simulink model "latesttopology1"  (R2014b)
settings: Solver=ode23tb  StartTime=0.0  StopTime=1  MaxStep=0.0001  MinStep=0.00001  RelTol=1e-3
libraries: powerlib x90, simulink x33, powerlib_meascontrol x2
settings Model: Creator=SELVA  LastModifiedBy=SELVA
settings DataIOCC: SignalLoggingSaveFormat=ModelDataLogs
settings OptimizationCC: ExpressionDepthLimit=2147483647
settings DebuggingCC: UnderspecifiedInitializationDetection=Classic  MergeDetectMultiDrivingBlocksExec=none  FcnCallInpInsideContextMsg=UseLocalSettings  StateNameClashWarn=warning
settings GRTTargetCC: CombineOutputUpdateFcns=off  GRTInterface=on

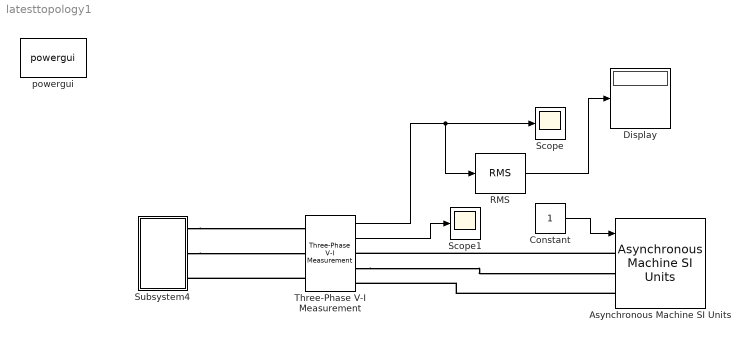
== system latesttopology1 ==
  Asynchronous Machine SI Units : powerlib/Machines/Asynchronous Machine SI Units  PresetModel="15:  5.4 HP (4KW)   400 V  50Hz 1430 RPM"  MechanicalLoad=Torque Tm  ShowDetailedParameters=on  RotorType=Squirrel-cage  ReferenceFrame=Rotor  Units=SI  MeasurementBus=off  NominalParameters=[4000 400 50]  Stator=[1.405 0.005839]  Rotor=[1.395 0.005839]  Cage1=[ 0.022 0.226/377]  Cage2=[ 0.022 0.226/377]  Lm=0.1722  Mechanical=[0.0131 0.002985 2]  PolePairs=2  InitialConditions=[1 0 0 0 0 0 0 0]  SimulateSaturation=off  Saturation=[14.03593122, 27.81365428, 53.79336849, 72.68890987, 97.98006896, 148.6815601, 215.7428561, 302.9841135, 420.4778367 ; 230, 322, 414, 460, 506, 552, 598, 644, 690]  LoadFlowParameters=1492000  TsPowergui=0  TsBlock=-1  IterativeModel=Trapezoidal non iterative  Pmec=0
  Constant : Constant
  Display : Display
  RMS : powerlib_meascontrol/Measurements/RMS  TrueRMS=on  Freq=50  RMSInit=0  Ts=0
  Scope : Scope
      settings: YMin=-800  YMax=800  SaveName=ScopeData3
  Scope1 : Scope
      settings: YMin=-800  YMax=800  SaveName=ScopeData4
  Subsystem4 : Subsystem  mask{v=66.5, fc=1000, m=1}
      mask prompts: v "DC Voltage"; fc "Switching Frequency"; m "Modulation Index"
  Three-Phase V-I Measurement : powerlib/Measurements/Three-Phase V-I Measurement  VoltageMeasurement=phase-to-ground  SetLabelV=off  LabelV=Vabc  Vpu=off  VpuLL=off  CurrentMeasurement=yes  SetLabelI=off  LabelI=Iabc  Ipu=off  Pbase=100e6  Vbase=500e3  OutputType=Complex  PhasorSimulation=off  PSBequivalent=0
  powergui : powerlib/powergui  Priority=1  SimulationMode=Discrete  SolverType=Tustin/Backward Euler (TBE)  SampleTime=50e-6  frequency=60  SPID=off  DisableSnubberDevices=off  DisableRonSwitches=off  DisableVfSwitches=off  SwTol=0  DisplayEquations=off  Interpol=off  methode=off  Ts=100  frequencyindice=0  Pbase=100e6  ErrMax=1e-4  Iterations=50  UnitsV=kV  UnitsW=MW  FunctionMessages=off  echomessages=off  HookPort=off  EnableUseOfTLC=off  x0status=blocks  RestoreLinks=warning  ResistiveCurrentMeasurement=off  Frange=[0:2:500]  Ylog=off  Xlog=on  ShowGrid=off  save=off  variable=ZData  structure=0  ZoomFFT=off  StartTime=0.0  cycles=1  DisplayStyle=1  fundamental=60  FreqAxis=off  MaxFrequency=1000  frequencyindicesteady=1  RmsSteady=1  display=off
  wires:
  Three-Phase V-I Measurement/1 -> RMS/1, Scope/1
  RMS/1 -> Display/1
  Three-Phase V-I Measurement/2 -> Scope1/1
  Constant/1 -> Asynchronous Machine SI Units/1
  connections:
  Asynchronous Machine SI Units/LConn1 -- Three-Phase V-I Measurement/RConn1
  Three-Phase V-I Measurement/RConn2 -- Asynchronous Machine SI Units/LConn2
  Asynchronous Machine SI Units/LConn3 -- Three-Phase V-I Measurement/RConn3
  Subsystem4/RConn1 -- Three-Phase V-I Measurement/LConn1
  Subsystem4/RConn2 -- Three-Phase V-I Measurement/LConn2
  Three-Phase V-I Measurement/LConn3 -- Subsystem4/RConn3

== system latesttopology1/Subsystem4 ==
  Ground : powerlib/Elements/Ground  LConnTagsString=a
  Subsystem1 : Subsystem
  Subsystem2 : Subsystem
  Subsystem3 : Subsystem
  A : PMIOPort  Port=1  Side=Right
  B : PMIOPort  Port=2  Side=Right
  C : PMIOPort  Port=3  Side=Right
  connections:
  Subsystem1/RConn2 -- Subsystem2/RConn2 -- Ground/LConn1 -- Subsystem3/RConn2
  B/RConn1 -- Subsystem2/RConn1
  A/RConn1 -- Subsystem1/RConn1
  Subsystem3/RConn1 -- C/RConn1

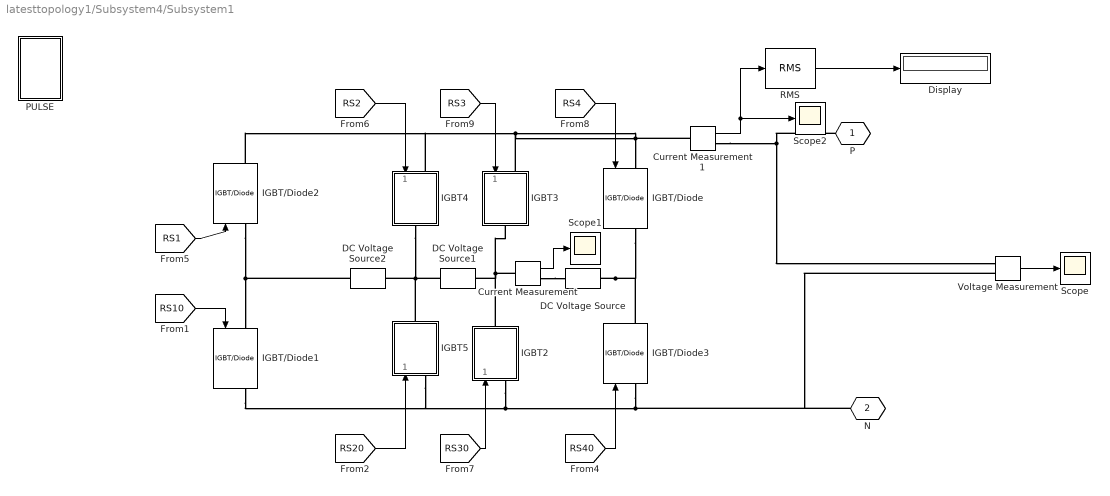
== system latesttopology1/Subsystem4/Subsystem1 ==
  Current Measurement : powerlib/Measurements/Current Measurement  PhasorSimulation=off  OutputType=Complex  PSBequivalent=0
  Current Measurement1 : powerlib/Measurements/Current Measurement  PhasorSimulation=off  OutputType=Complex  PSBequivalent=0
  DC Voltage Source : powerlib/Electrical Sources/DC Voltage Source  Amplitude=v  Measurements=None
  DC Voltage Source1 : powerlib/Electrical Sources/DC Voltage Source  Amplitude=2*v  Measurements=None
  DC Voltage Source2 : powerlib/Electrical Sources/DC Voltage Source  Amplitude=2*v  Measurements=None
  Display : Display
  IGBT/Diode{,1..3} (4 alike) : powerlib/Power Electronics/IGBT//Diode  Ron=1e-3  Rs=1e5  Cs=inf  Measurements=on
  IGBT2 : Subsystem
  IGBT3 : Subsystem
  IGBT4 : Subsystem
  IGBT5 : Subsystem
  PULSE : Subsystem
  RMS : powerlib_meascontrol/Measurements/RMS  TrueRMS=on  Freq=50  RMSInit=120  Ts=0
  Scope : Scope
      settings: YMin=-50  YMax=50  SaveName=ScopeData2
  Scope1 : Scope
      settings: YMin=-50  YMax=50  SaveName=ScopeData5
  Scope2 : Scope
      settings: YMin=-6  YMax=8  SaveName=ScopeData6
  Voltage Measurement : powerlib/Measurements/Voltage Measurement  PhasorSimulation=off  OutputType=Complex  PSBequivalent=0
  P : PMIOPort  Port=1  Side=Right
  N : PMIOPort  Port=2  Side=Right
  wires:
  Voltage Measurement/1 -> Scope/1
  [RS1] -> IGBT/Diode2/1
  [RS4] -> IGBT/Diode/1
  [RS10] -> IGBT/Diode1/1
  [RS40] -> IGBT/Diode3/1
  [RS2] -> IGBT4/1(Gate)
  [RS3] -> IGBT3/1(Gate)
  [RS20] -> IGBT5/1(Gate)
  [RS30] -> IGBT2/1(Gate)
  Current Measurement/1 -> Scope1/1
  Current Measurement1/1 -> Scope2/1, RMS/1
  RMS/1 -> Display/1
  connections:
  DC Voltage Source1/RConn1 -- IGBT4/RConn1 -- IGBT5/RConn1 -- DC Voltage Source2/LConn1
  IGBT2/RConn1 -- DC Voltage Source1/LConn1 -- Current Measurement/LConn1 -- IGBT3/RConn1
  IGBT3/LConn1 -- IGBT4/LConn1 -- IGBT/Diode2/RConn1 -- Current Measurement1/LConn1 -- IGBT/Diode/LConn1
  IGBT2/LConn1 -- IGBT5/LConn1 -- IGBT/Diode1/RConn1 -- Voltage Measurement/LConn2 -- N/RConn1 -- IGBT/Diode3/LConn1
  DC Voltage Source/LConn1 -- IGBT/Diode3/RConn1 -- IGBT/Diode/RConn1
  IGBT/Diode2/LConn1 -- DC Voltage Source2/RConn1 -- IGBT/Diode1/LConn1
  Current Measurement/RConn1 -- DC Voltage Source/RConn1
  P/RConn1 -- Current Measurement1/RConn1 -- Voltage Measurement/LConn1

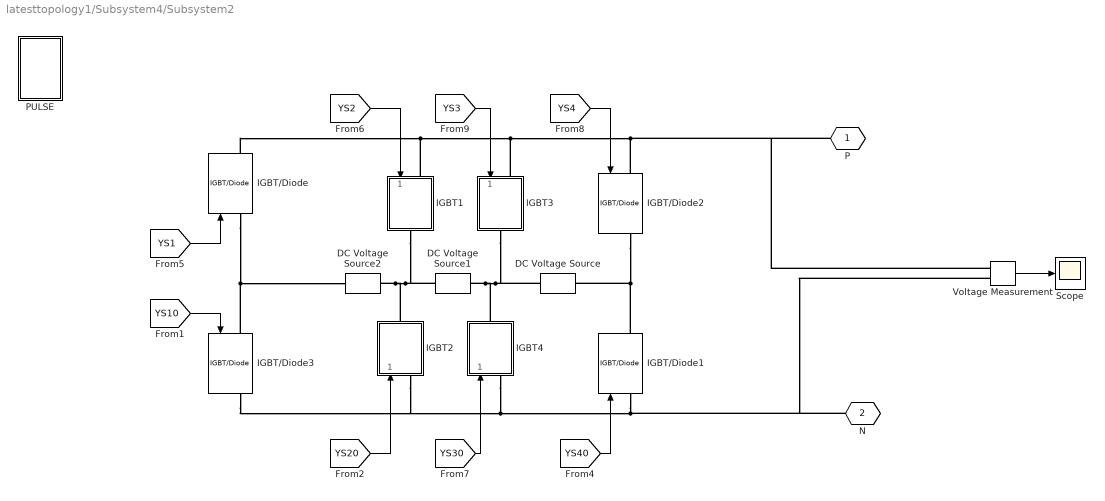
== system latesttopology1/Subsystem4/Subsystem2 ==
  DC Voltage Source : powerlib/Electrical Sources/DC Voltage Source  Amplitude=v  Measurements=None
  DC Voltage Source1 : powerlib/Electrical Sources/DC Voltage Source  Amplitude=2*v  Measurements=None
  DC Voltage Source2 : powerlib/Electrical Sources/DC Voltage Source  Amplitude=2*v  Measurements=None
  IGBT/Diode{,1..3} (4 alike) : powerlib/Power Electronics/IGBT//Diode  Ron=1e-3  Rs=1e5  Cs=inf  Measurements=on
  IGBT1 : Subsystem
  IGBT2 : Subsystem
  IGBT3 : Subsystem
  IGBT4 : Subsystem
  PULSE : Subsystem
  Scope : Scope
      settings: YMin=-50  YMax=50
  Voltage Measurement : powerlib/Measurements/Voltage Measurement  PhasorSimulation=off  OutputType=Complex  PSBequivalent=0
  P : PMIOPort  Port=1  Side=Right
  N : PMIOPort  Port=2  Side=Right
  wires:
  [YS30] -> IGBT4/1(Gate)
  [YS20] -> IGBT2/1(Gate)
  [YS3] -> IGBT3/1(Gate)
  [YS2] -> IGBT1/1(Gate)
  [YS40] -> IGBT/Diode1/1
  [YS10] -> IGBT/Diode3/1
  [YS4] -> IGBT/Diode2/1
  [YS1] -> IGBT/Diode/1
  Voltage Measurement/1 -> Scope/1
  connections:
  IGBT/Diode3/LConn1 -- IGBT/Diode/LConn1 -- DC Voltage Source2/RConn1
  IGBT/Diode2/RConn1 -- IGBT/Diode1/RConn1 -- DC Voltage Source/LConn1
  IGBT/Diode1/LConn1 -- N/RConn1 -- Voltage Measurement/LConn2 -- IGBT2/LConn1 -- IGBT/Diode3/RConn1 -- IGBT4/LConn1
  IGBT/Diode/RConn1 -- IGBT3/LConn1 -- IGBT/Diode2/LConn1 -- P/RConn1 -- Voltage Measurement/LConn1 -- IGBT1/LConn1
  DC Voltage Source1/LConn1 -- IGBT3/RConn1 -- DC Voltage Source/RConn1 -- IGBT4/RConn1
  DC Voltage Source2/LConn1 -- IGBT1/RConn1 -- DC Voltage Source1/RConn1 -- IGBT2/RConn1

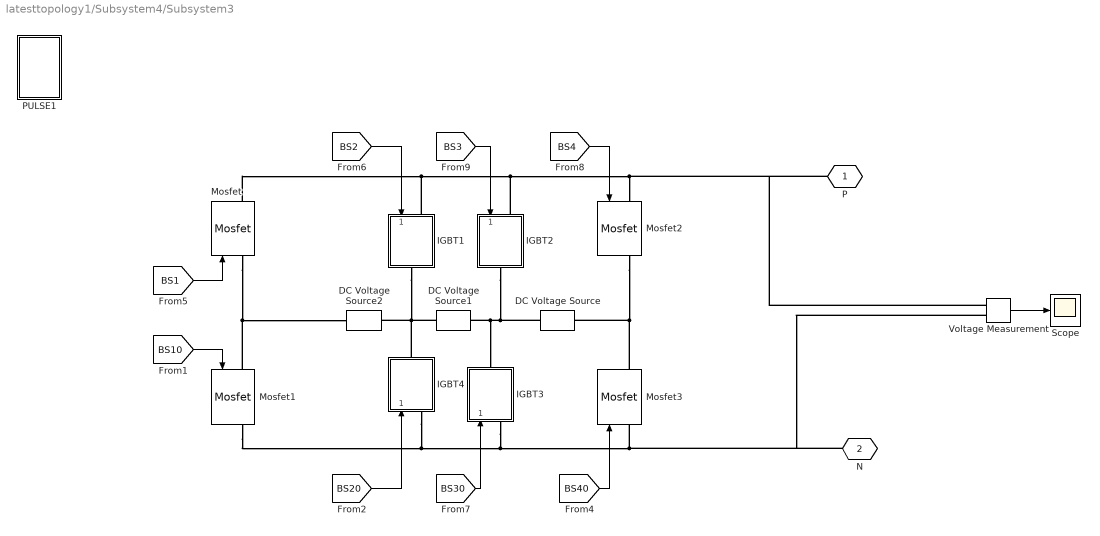
== system latesttopology1/Subsystem4/Subsystem3 ==
  DC Voltage Source : powerlib/Electrical Sources/DC Voltage Source  Amplitude=v  Measurements=None
  DC Voltage Source1 : powerlib/Electrical Sources/DC Voltage Source  Amplitude=2*v  Measurements=None
  DC Voltage Source2 : powerlib/Electrical Sources/DC Voltage Source  Amplitude=2*v  Measurements=None
  IGBT1 : Subsystem
  IGBT2 : Subsystem
  IGBT3 : Subsystem
  IGBT4 : Subsystem
  Mosfet{,1..3} (4 alike) : powerlib/Power Electronics/Mosfet  Ron=0.1  Lon=0  Rd=0.01  Vfd=0  IC=0  Rs=1e5  Cs=inf  Measurements=on
  PULSE1 : Subsystem
  Scope : Scope
      settings: YMin=-50  YMax=50
  Voltage Measurement : powerlib/Measurements/Voltage Measurement  PhasorSimulation=off  OutputType=Complex  PSBequivalent=0
  P : PMIOPort  Port=1  Side=Right
  N : PMIOPort  Port=2  Side=Right
  wires:
  Voltage Measurement/1 -> Scope/1
  [BS1] -> Mosfet/1
  [BS4] -> Mosfet2/1
  [BS10] -> Mosfet1/1
  [BS40] -> Mosfet3/1
  [BS2] -> IGBT1/1(Gate)
  [BS3] -> IGBT2/1(Gate)
  [BS20] -> IGBT4/1(Gate)
  [BS30] -> IGBT3/1(Gate)
  connections:
  IGBT4/RConn1 -- IGBT1/RConn1 -- DC Voltage Source1/RConn1 -- DC Voltage Source2/LConn1
  IGBT2/RConn1 -- DC Voltage Source/RConn1 -- IGBT3/RConn1 -- DC Voltage Source1/LConn1
  IGBT1/LConn1 -- IGBT2/LConn1 -- Voltage Measurement/LConn1 -- P/RConn1 -- Mosfet2/LConn1 -- Mosfet/RConn1
  Mosfet1/RConn1 -- IGBT4/LConn1 -- Voltage Measurement/LConn2 -- N/RConn1 -- Mosfet3/LConn1 -- IGBT3/LConn1
  Mosfet2/RConn1 -- DC Voltage Source/LConn1 -- Mosfet3/RConn1
  Mosfet/LConn1 -- Mosfet1/LConn1 -- DC Voltage Source2/RConn1

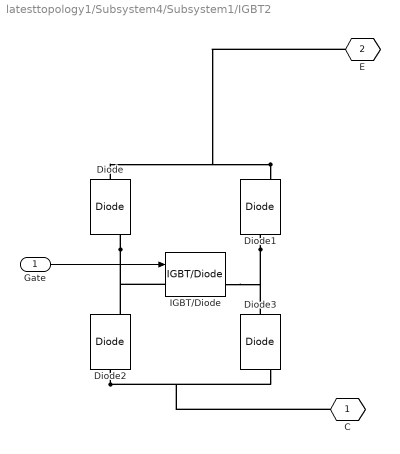
== system latesttopology1/Subsystem4/Subsystem1/IGBT2 ==
  Gate : Inport
  Diode{,1..3} (4 alike) : powerlib/Power Electronics/Diode  Ron=0.001  Lon=0  Vf=0.8  IC=0  UseSnubber=off  Rs=500  Cs=250e-9  Measurements=on
  IGBT/Diode : powerlib/Power Electronics/IGBT//Diode  Ron=1e-3  Rs=1e5  Cs=inf  Measurements=on
  C : PMIOPort  Port=1  Side=Left
  E : PMIOPort  Port=2  Side=Right
  wires:
  Gate/1 -> IGBT/Diode/1
  connections:
  Diode/RConn1 -- Diode2/RConn1 -- IGBT/Diode/LConn1
  Diode1/LConn1 -- Diode3/LConn1 -- IGBT/Diode/RConn1
  Diode2/LConn1 -- Diode3/RConn1 -- C/RConn1
  Diode1/RConn1 -- Diode/LConn1 -- E/RConn1

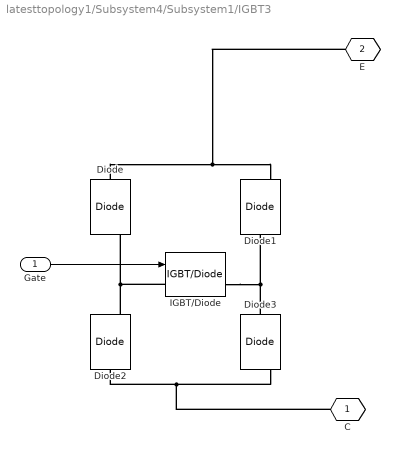
== system latesttopology1/Subsystem4/Subsystem1/IGBT3 ==
  Gate : Inport
  Diode{,1..3} (4 alike) : powerlib/Power Electronics/Diode  Ron=0.001  Lon=0  Vf=0.8  IC=0  UseSnubber=off  Rs=500  Cs=250e-9  Measurements=on
  IGBT/Diode : powerlib/Power Electronics/IGBT//Diode  Ron=1e-3  Rs=1e5  Cs=inf  Measurements=on
  C : PMIOPort  Port=1  Side=Left
  E : PMIOPort  Port=2  Side=Right
  wires:
  Gate/1 -> IGBT/Diode/1
  connections:
  E/RConn1 -- Diode/LConn1 -- Diode1/RConn1
  C/RConn1 -- Diode3/RConn1 -- Diode2/LConn1
  IGBT/Diode/RConn1 -- Diode3/LConn1 -- Diode1/LConn1
  IGBT/Diode/LConn1 -- Diode2/RConn1 -- Diode/RConn1

== system latesttopology1/Subsystem4/Subsystem1/IGBT4 ==
  Gate : Inport
  Diode{,1..3} (4 alike) : powerlib/Power Electronics/Diode  Ron=0.001  Lon=0  Vf=0.8  IC=0  UseSnubber=off  Rs=500  Cs=250e-9  Measurements=on
  IGBT/Diode : powerlib/Power Electronics/IGBT//Diode  Ron=1e-3  Rs=1e5  Cs=inf  Measurements=on
  C : PMIOPort  Port=1  Side=Left
  E : PMIOPort  Port=2  Side=Right
  wires:
  Gate/1 -> IGBT/Diode/1
  connections:
  Diode/RConn1 -- Diode2/RConn1 -- IGBT/Diode/LConn1
  Diode1/LConn1 -- Diode3/LConn1 -- IGBT/Diode/RConn1
  Diode2/LConn1 -- Diode3/RConn1 -- C/RConn1
  Diode1/RConn1 -- Diode/LConn1 -- E/RConn1

== system latesttopology1/Subsystem4/Subsystem1/IGBT5 ==
  Gate : Inport
  Diode{,1..3} (4 alike) : powerlib/Power Electronics/Diode  Ron=0.001  Lon=0  Vf=0.8  IC=0  UseSnubber=off  Rs=500  Cs=250e-9  Measurements=on
  IGBT/Diode : powerlib/Power Electronics/IGBT//Diode  Ron=1e-3  Rs=1e5  Cs=inf  Measurements=on
  C : PMIOPort  Port=1  Side=Left
  E : PMIOPort  Port=2  Side=Right
  wires:
  Gate/1 -> IGBT/Diode/1
  connections:
  E/RConn1 -- Diode/LConn1 -- Diode1/RConn1
  C/RConn1 -- Diode3/RConn1 -- Diode2/LConn1
  IGBT/Diode/RConn1 -- Diode3/LConn1 -- Diode1/LConn1
  IGBT/Diode/LConn1 -- Diode2/RConn1 -- Diode/RConn1

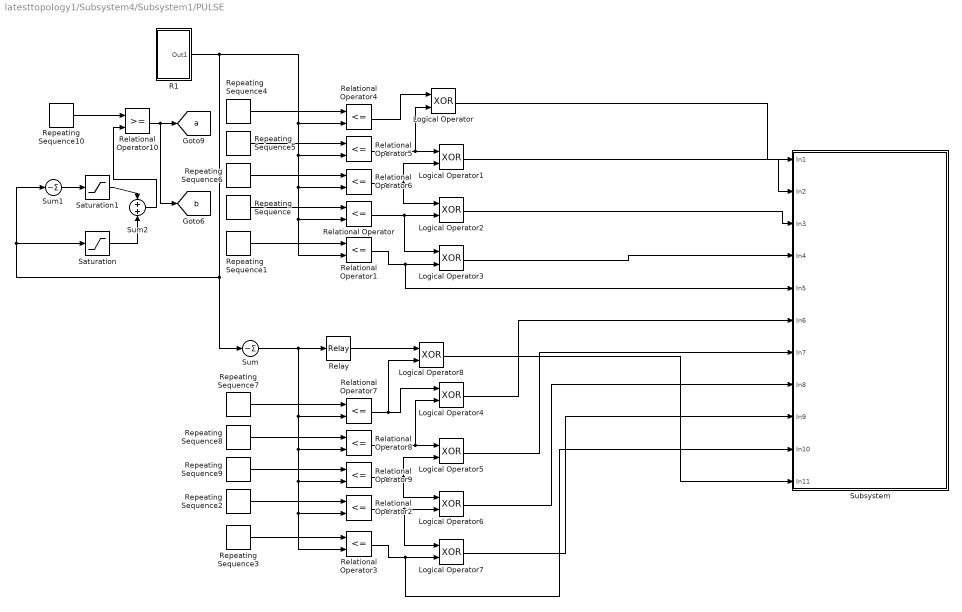
== system latesttopology1/Subsystem4/Subsystem1/PULSE ==
  Logical Operator{,1..8} (9 alike) : Logic  Operator=XOR  AllPortsSameDT=off  OutDataTypeStr=boolean
  R1 : Subsystem
  Relational Operator{,1..9} (10 alike) : RelationalOperator  Operator=<=  OutDataTypeStr=boolean
  Relational Operator10 : RelationalOperator  OutDataTypeStr=boolean
  Relay : Relay  OnOutputValue=0  OffOutputValue=1
  Repeating Sequence : simulink/Sources/Repeating Sequence  rep_seq_t="[0 (1/fc)/2  (1/fc)]"  rep_seq_y=[3/5 4/5 3/5]
  Repeating Sequence1 : simulink/Sources/Repeating Sequence  rep_seq_t="[0 (1/fc)/2  (1/fc)]"  rep_seq_y=[4/5 1 4/5]
  Repeating Sequence10 : simulink/Sources/Repeating Sequence  rep_seq_t="[0 (1/fc)/2  (1/fc)]"  rep_seq_y=[0 1/5 0]
  Repeating Sequence2 : simulink/Sources/Repeating Sequence  rep_seq_t="[0 (1/fc)/2  (1/fc)]"  rep_seq_y=[3/5 4/5 3/5]
  Repeating Sequence3 : simulink/Sources/Repeating Sequence  rep_seq_t="[0 (1/fc)/2  (1/fc)]"  rep_seq_y=[4/5 1 4/5]
  Repeating Sequence4 : simulink/Sources/Repeating Sequence  rep_seq_t="[0 (1/fc)/2  (1/fc)]"  rep_seq_y=[0 1/5 0]
  Repeating Sequence5 : simulink/Sources/Repeating Sequence  rep_seq_t="[0 (1/fc)/2  (1/fc)]"  rep_seq_y=[1/5 2/5 1/5]
  Repeating Sequence6 : simulink/Sources/Repeating Sequence  rep_seq_t="[0 (1/fc)/2  (1/fc)]"  rep_seq_y=[2/5 3/5 2/5]
  Repeating Sequence7 : simulink/Sources/Repeating Sequence  rep_seq_t="[0 (1/fc)/2  (1/fc)]"  rep_seq_y=[0 1/5 0]
  Repeating Sequence8 : simulink/Sources/Repeating Sequence  rep_seq_t="[0 (1/fc)/2  (1/fc)]"  rep_seq_y=[1/5 2/5 1/5]
  Repeating Sequence9 : simulink/Sources/Repeating Sequence  rep_seq_t="[0 (1/fc)/2  (1/fc)]"  rep_seq_y=[2/5 3/5 2/5]
  Saturation : Saturate  UpperLimit=1  LowerLimit=0
  Saturation1 : Saturate  UpperLimit=1  LowerLimit=0
  Subsystem : Subsystem
  Sum : Sum  Inputs=-
  Sum1 : Sum  Inputs=-
  Sum2 : Sum
  tag scope: a=global, b=global
  wires:
  Repeating Sequence1/1 -> Relational Operator1/1
  Repeating Sequence/1 -> Relational Operator/1
  Repeating Sequence6/1 -> Relational Operator6/1
  Repeating Sequence5/1 -> Relational Operator5/1
  Repeating Sequence4/1 -> Relational Operator4/1
  R1/1(Out1) -> Sum1/1, Saturation/1, Sum/1, Relational Operator4/2, Relational Operator5/2, Relational Operator6/2, Relational Operator1/2, Relational Operator/2
  Relational Operator4/1 -> Logical Operator/1
  Relational Operator5/1 -> Logical Operator1/1, Logical Operator/2
  Relational Operator6/1 -> Logical Operator2/1, Logical Operator1/2
  Relational Operator/1 -> Logical Operator3/1, Logical Operator2/2
  Relational Operator1/1 -> Subsystem/5(In5), Logical Operator3/2
  Repeating Sequence3/1 -> Relational Operator3/1
  Repeating Sequence2/1 -> Relational Operator2/1
  Repeating Sequence9/1 -> Relational Operator9/1
  Repeating Sequence8/1 -> Relational Operator8/1
  Repeating Sequence7/1 -> Relational Operator7/1
  Sum/1 -> Relay/1, Relational Operator7/2, Relational Operator8/2, Relational Operator9/2, Relational Operator3/2, Relational Operator2/2
  Relational Operator7/1 -> Logical Operator8/2, Logical Operator4/1
  Relational Operator8/1 -> Logical Operator5/1, Logical Operator4/2
  Relational Operator9/1 -> Logical Operator6/1, Logical Operator5/2
  Relational Operator2/1 -> Logical Operator7/1, Logical Operator6/2
  Relational Operator3/1 -> Subsystem/10(In10), Logical Operator7/2
  Logical Operator4/1 -> Subsystem/6(In6)
  Logical Operator6/1 -> Subsystem/8(In8)
  Logical Operator7/1 -> Subsystem/9(In9)
  Logical Operator/1 -> Subsystem/1(In1)
  Logical Operator1/1 -> Subsystem/2(In2)
  Logical Operator2/1 -> Subsystem/3(In3)
  Logical Operator3/1 -> Subsystem/4(In4)
  Logical Operator5/1 -> Subsystem/7(In7)
  Relay/1 -> Logical Operator8/1
  Logical Operator8/1 -> Subsystem/11(In11)
  Sum1/1 -> Saturation1/1
  Saturation1/1 -> Sum2/1
  Saturation/1 -> Sum2/2
  Repeating Sequence10/1 -> Relational Operator10/1
  Sum2/1 -> Relational Operator10/2
  Relational Operator10/1 -> [b], [a]

== system latesttopology1/Subsystem4/Subsystem2/IGBT1 ==
  Gate : Inport
  Diode{,1..3} (4 alike) : powerlib/Power Electronics/Diode  Ron=0.001  Lon=0  Vf=0.8  IC=0  UseSnubber=off  Rs=500  Cs=250e-9  Measurements=on
  IGBT/Diode : powerlib/Power Electronics/IGBT//Diode  Ron=1e-3  Rs=1e5  Cs=inf  Measurements=on
  C : PMIOPort  Port=1  Side=Left
  E : PMIOPort  Port=2  Side=Right
  wires:
  Gate/1 -> IGBT/Diode/1
  connections:
  Diode/RConn1 -- Diode2/RConn1 -- IGBT/Diode/LConn1
  Diode1/LConn1 -- Diode3/LConn1 -- IGBT/Diode/RConn1
  Diode2/LConn1 -- Diode3/RConn1 -- C/RConn1
  Diode1/RConn1 -- Diode/LConn1 -- E/RConn1

== system latesttopology1/Subsystem4/Subsystem2/IGBT2 ==
  Gate : Inport
  Diode{,1..3} (4 alike) : powerlib/Power Electronics/Diode  Ron=0.001  Lon=0  Vf=0.8  IC=0  UseSnubber=off  Rs=500  Cs=250e-9  Measurements=on
  IGBT/Diode : powerlib/Power Electronics/IGBT//Diode  Ron=1e-3  Rs=1e5  Cs=inf  Measurements=on
  C : PMIOPort  Port=1  Side=Left
  E : PMIOPort  Port=2  Side=Right
  wires:
  Gate/1 -> IGBT/Diode/1
  connections:
  E/RConn1 -- Diode/LConn1 -- Diode1/RConn1
  C/RConn1 -- Diode3/RConn1 -- Diode2/LConn1
  IGBT/Diode/RConn1 -- Diode3/LConn1 -- Diode1/LConn1
  IGBT/Diode/LConn1 -- Diode2/RConn1 -- Diode/RConn1

== system latesttopology1/Subsystem4/Subsystem2/IGBT3 ==
  Gate : Inport
  Diode{,1..3} (4 alike) : powerlib/Power Electronics/Diode  Ron=0.001  Lon=0  Vf=0.8  IC=0  UseSnubber=off  Rs=500  Cs=250e-9  Measurements=on
  IGBT/Diode : powerlib/Power Electronics/IGBT//Diode  Ron=1e-3  Rs=1e5  Cs=inf  Measurements=on
  C : PMIOPort  Port=1  Side=Left
  E : PMIOPort  Port=2  Side=Right
  wires:
  Gate/1 -> IGBT/Diode/1
  connections:
  E/RConn1 -- Diode/LConn1 -- Diode1/RConn1
  C/RConn1 -- Diode3/RConn1 -- Diode2/LConn1
  IGBT/Diode/RConn1 -- Diode3/LConn1 -- Diode1/LConn1
  IGBT/Diode/LConn1 -- Diode2/RConn1 -- Diode/RConn1

== system latesttopology1/Subsystem4/Subsystem2/IGBT4 ==
  Gate : Inport
  Diode{,1..3} (4 alike) : powerlib/Power Electronics/Diode  Ron=0.001  Lon=0  Vf=0.8  IC=0  UseSnubber=off  Rs=500  Cs=250e-9  Measurements=on
  IGBT/Diode : powerlib/Power Electronics/IGBT//Diode  Ron=1e-3  Rs=1e5  Cs=inf  Measurements=on
  C : PMIOPort  Port=1  Side=Left
  E : PMIOPort  Port=2  Side=Right
  wires:
  Gate/1 -> IGBT/Diode/1
  connections:
  Diode/RConn1 -- Diode2/RConn1 -- IGBT/Diode/LConn1
  Diode1/LConn1 -- Diode3/LConn1 -- IGBT/Diode/RConn1
  Diode2/LConn1 -- Diode3/RConn1 -- C/RConn1
  Diode1/RConn1 -- Diode/LConn1 -- E/RConn1

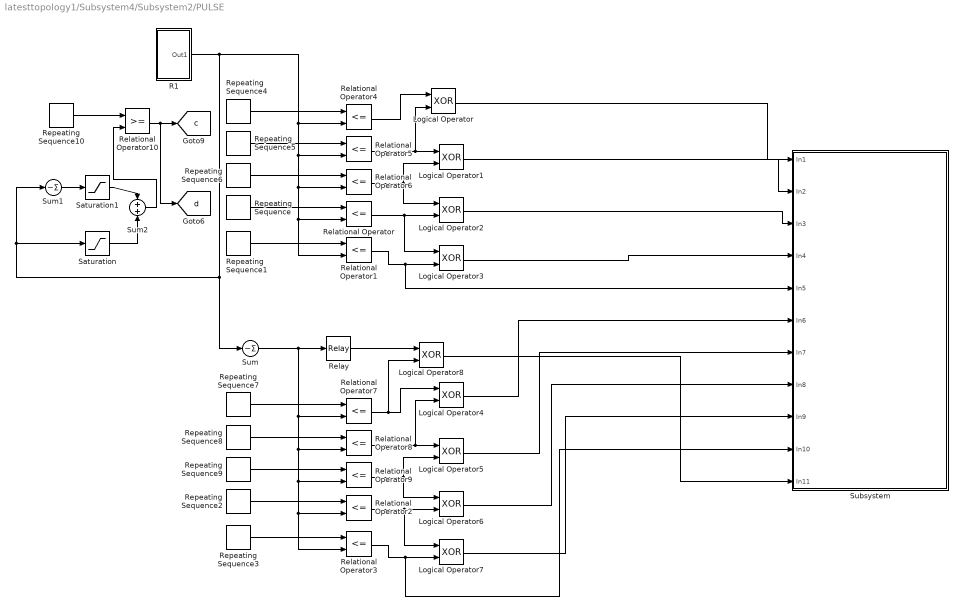
== system latesttopology1/Subsystem4/Subsystem2/PULSE ==
  Logical Operator{,1..8} (9 alike) : Logic  Operator=XOR  AllPortsSameDT=off  OutDataTypeStr=boolean
  R1 : Subsystem
  Relational Operator{,1..9} (10 alike) : RelationalOperator  Operator=<=  OutDataTypeStr=boolean
  Relational Operator10 : RelationalOperator  OutDataTypeStr=boolean
  Relay : Relay  OnOutputValue=0  OffOutputValue=1
  Repeating Sequence : simulink/Sources/Repeating Sequence  rep_seq_t="[0 (1/fc)/2  (1/fc)]"  rep_seq_y=[3/5 4/5 3/5]
  Repeating Sequence1 : simulink/Sources/Repeating Sequence  rep_seq_t="[0 (1/fc)/2  (1/fc)]"  rep_seq_y=[4/5 1 4/5]
  Repeating Sequence10 : simulink/Sources/Repeating Sequence  rep_seq_t="[0 (1/fc)/2  (1/fc)]"  rep_seq_y=[0 1/5 0]
  Repeating Sequence2 : simulink/Sources/Repeating Sequence  rep_seq_t="[0 (1/fc)/2  (1/fc)]"  rep_seq_y=[3/5 4/5 3/5]
  Repeating Sequence3 : simulink/Sources/Repeating Sequence  rep_seq_t="[0 (1/fc)/2  (1/fc)]"  rep_seq_y=[4/5 1 4/5]
  Repeating Sequence4 : simulink/Sources/Repeating Sequence  rep_seq_t="[0 (1/fc)/2  (1/fc)]"  rep_seq_y=[0 1/5 0]
  Repeating Sequence5 : simulink/Sources/Repeating Sequence  rep_seq_t="[0 (1/fc)/2  (1/fc)]"  rep_seq_y=[1/5 2/5 1/5]
  Repeating Sequence6 : simulink/Sources/Repeating Sequence  rep_seq_t="[0 (1/fc)/2  (1/fc)]"  rep_seq_y=[2/5 3/5 2/5]
  Repeating Sequence7 : simulink/Sources/Repeating Sequence  rep_seq_t="[0 (1/fc)/2  (1/fc)]"  rep_seq_y=[0 1/5 0]
  Repeating Sequence8 : simulink/Sources/Repeating Sequence  rep_seq_t="[0 (1/fc)/2  (1/fc)]"  rep_seq_y=[1/5 2/5 1/5]
  Repeating Sequence9 : simulink/Sources/Repeating Sequence  rep_seq_t="[0 (1/fc)/2  (1/fc)]"  rep_seq_y=[2/5 3/5 2/5]
  Saturation : Saturate  UpperLimit=1  LowerLimit=0
  Saturation1 : Saturate  UpperLimit=1  LowerLimit=0
  Subsystem : Subsystem
  Sum : Sum  Inputs=-
  Sum1 : Sum  Inputs=-
  Sum2 : Sum
  tag scope: c=global, d=global
  wires:
  Relational Operator10/1 -> [c], [d]
  Sum2/1 -> Relational Operator10/2
  Repeating Sequence10/1 -> Relational Operator10/1
  Saturation/1 -> Sum2/2
  Saturation1/1 -> Sum2/1
  Sum1/1 -> Saturation1/1
  Logical Operator8/1 -> Subsystem/11(In11)
  Relay/1 -> Logical Operator8/1
  Logical Operator5/1 -> Subsystem/7(In7)
  Logical Operator3/1 -> Subsystem/4(In4)
  Logical Operator2/1 -> Subsystem/3(In3)
  Logical Operator1/1 -> Subsystem/2(In2)
  Logical Operator/1 -> Subsystem/1(In1)
  Logical Operator7/1 -> Subsystem/9(In9)
  Logical Operator6/1 -> Subsystem/8(In8)
  Logical Operator4/1 -> Subsystem/6(In6)
  Relational Operator3/1 -> Logical Operator7/2, Subsystem/10(In10)
  Relational Operator2/1 -> Logical Operator6/2, Logical Operator7/1
  Relational Operator9/1 -> Logical Operator5/2, Logical Operator6/1
  Relational Operator8/1 -> Logical Operator4/2, Logical Operator5/1
  Relational Operator7/1 -> Logical Operator4/1, Logical Operator8/2
  Sum/1 -> Relational Operator2/2, Relational Operator3/2, Relational Operator9/2, Relational Operator8/2, Relational Operator7/2, Relay/1
  Repeating Sequence7/1 -> Relational Operator7/1
  Repeating Sequence8/1 -> Relational Operator8/1
  Repeating Sequence9/1 -> Relational Operator9/1
  Repeating Sequence2/1 -> Relational Operator2/1
  Repeating Sequence3/1 -> Relational Operator3/1
  Relational Operator1/1 -> Logical Operator3/2, Subsystem/5(In5)
  Relational Operator/1 -> Logical Operator2/2, Logical Operator3/1
  Relational Operator6/1 -> Logical Operator1/2, Logical Operator2/1
  Relational Operator5/1 -> Logical Operator/2, Logical Operator1/1
  Relational Operator4/1 -> Logical Operator/1
  R1/1(Out1) -> Relational Operator/2, Relational Operator1/2, Relational Operator6/2, Relational Operator5/2, Relational Operator4/2, Sum/1, Saturation/1, Sum1/1
  Repeating Sequence4/1 -> Relational Operator4/1
  Repeating Sequence5/1 -> Relational Operator5/1
  Repeating Sequence6/1 -> Relational Operator6/1
  Repeating Sequence/1 -> Relational Operator/1
  Repeating Sequence1/1 -> Relational Operator1/1

== system latesttopology1/Subsystem4/Subsystem3/IGBT1 ==
  Gate : Inport
  Diode{,1..3} (4 alike) : powerlib/Power Electronics/Diode  Ron=0.001  Lon=0  Vf=0.8  IC=0  UseSnubber=off  Rs=500  Cs=250e-9  Measurements=on
  IGBT/Diode : powerlib/Power Electronics/IGBT//Diode  Ron=1e-3  Rs=1e5  Cs=inf  Measurements=on
  C : PMIOPort  Port=1  Side=Left
  E : PMIOPort  Port=2  Side=Right
  wires:
  Gate/1 -> IGBT/Diode/1
  connections:
  E/RConn1 -- Diode/LConn1 -- Diode1/RConn1
  C/RConn1 -- Diode3/RConn1 -- Diode2/LConn1
  IGBT/Diode/RConn1 -- Diode3/LConn1 -- Diode1/LConn1
  IGBT/Diode/LConn1 -- Diode2/RConn1 -- Diode/RConn1

== system latesttopology1/Subsystem4/Subsystem3/IGBT2 ==
  Gate : Inport
  Diode{,1..3} (4 alike) : powerlib/Power Electronics/Diode  Ron=0.001  Lon=0  Vf=0.8  IC=0  UseSnubber=off  Rs=500  Cs=250e-9  Measurements=on
  IGBT/Diode : powerlib/Power Electronics/IGBT//Diode  Ron=1e-3  Rs=1e5  Cs=inf  Measurements=on
  C : PMIOPort  Port=1  Side=Left
  E : PMIOPort  Port=2  Side=Right
  wires:
  Gate/1 -> IGBT/Diode/1
  connections:
  Diode/RConn1 -- Diode2/RConn1 -- IGBT/Diode/LConn1
  Diode1/LConn1 -- Diode3/LConn1 -- IGBT/Diode/RConn1
  Diode2/LConn1 -- Diode3/RConn1 -- C/RConn1
  Diode1/RConn1 -- Diode/LConn1 -- E/RConn1

== system latesttopology1/Subsystem4/Subsystem3/IGBT3 ==
  Gate : Inport
  Diode{,1..3} (4 alike) : powerlib/Power Electronics/Diode  Ron=0.001  Lon=0  Vf=0.8  IC=0  UseSnubber=off  Rs=500  Cs=250e-9  Measurements=on
  IGBT/Diode : powerlib/Power Electronics/IGBT//Diode  Ron=1e-3  Rs=1e5  Cs=inf  Measurements=on
  C : PMIOPort  Port=1  Side=Left
  E : PMIOPort  Port=2  Side=Right
  wires:
  Gate/1 -> IGBT/Diode/1
  connections:
  E/RConn1 -- Diode/LConn1 -- Diode1/RConn1
  C/RConn1 -- Diode3/RConn1 -- Diode2/LConn1
  IGBT/Diode/RConn1 -- Diode3/LConn1 -- Diode1/LConn1
  IGBT/Diode/LConn1 -- Diode2/RConn1 -- Diode/RConn1

== system latesttopology1/Subsystem4/Subsystem3/IGBT4 ==
  Gate : Inport
  Diode{,1..3} (4 alike) : powerlib/Power Electronics/Diode  Ron=0.001  Lon=0  Vf=0.8  IC=0  UseSnubber=off  Rs=500  Cs=250e-9  Measurements=on
  IGBT/Diode : powerlib/Power Electronics/IGBT//Diode  Ron=1e-3  Rs=1e5  Cs=inf  Measurements=on
  C : PMIOPort  Port=1  Side=Left
  E : PMIOPort  Port=2  Side=Right
  wires:
  Gate/1 -> IGBT/Diode/1
  connections:
  Diode/RConn1 -- Diode2/RConn1 -- IGBT/Diode/LConn1
  Diode1/LConn1 -- Diode3/LConn1 -- IGBT/Diode/RConn1
  Diode2/LConn1 -- Diode3/RConn1 -- C/RConn1
  Diode1/RConn1 -- Diode/LConn1 -- E/RConn1

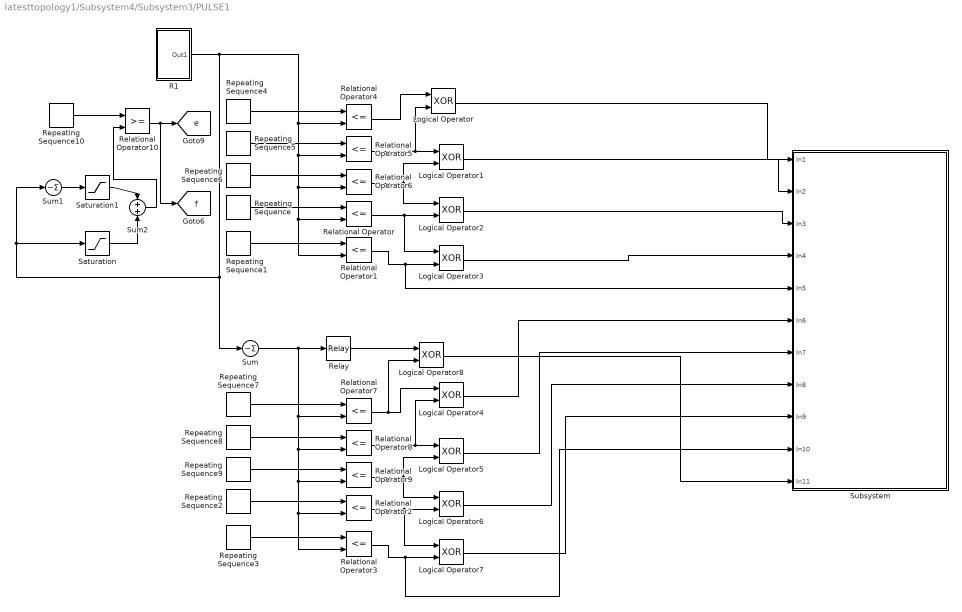
== system latesttopology1/Subsystem4/Subsystem3/PULSE1 ==
  Logical Operator{,1..8} (9 alike) : Logic  Operator=XOR  AllPortsSameDT=off  OutDataTypeStr=boolean
  R1 : Subsystem
  Relational Operator{,1..9} (10 alike) : RelationalOperator  Operator=<=  OutDataTypeStr=boolean
  Relational Operator10 : RelationalOperator  OutDataTypeStr=boolean
  Relay : Relay  OnOutputValue=0  OffOutputValue=1
  Repeating Sequence : simulink/Sources/Repeating Sequence  rep_seq_t="[0 (1/fc)/2  (1/fc)]"  rep_seq_y=[3/5 4/5 3/5]
  Repeating Sequence1 : simulink/Sources/Repeating Sequence  rep_seq_t="[0 (1/fc)/2  (1/fc)]"  rep_seq_y=[4/5 1 4/5]
  Repeating Sequence10 : simulink/Sources/Repeating Sequence  rep_seq_t="[0 (1/fc)/2  (1/fc)]"  rep_seq_y=[0 1/5 0]
  Repeating Sequence2 : simulink/Sources/Repeating Sequence  rep_seq_t="[0 (1/fc)/2  (1/fc)]"  rep_seq_y=[3/5 4/5 3/5]
  Repeating Sequence3 : simulink/Sources/Repeating Sequence  rep_seq_t="[0 (1/fc)/2  (1/fc)]"  rep_seq_y=[4/5 1 4/5]
  Repeating Sequence4 : simulink/Sources/Repeating Sequence  rep_seq_t="[0 (1/fc)/2  (1/fc)]"  rep_seq_y=[0 1/5 0]
  Repeating Sequence5 : simulink/Sources/Repeating Sequence  rep_seq_t="[0 (1/fc)/2  (1/fc)]"  rep_seq_y=[1/5 2/5 1/5]
  Repeating Sequence6 : simulink/Sources/Repeating Sequence  rep_seq_t="[0 (1/fc)/2  (1/fc)]"  rep_seq_y=[2/5 3/5 2/5]
  Repeating Sequence7 : simulink/Sources/Repeating Sequence  rep_seq_t="[0 (1/fc)/2  (1/fc)]"  rep_seq_y=[0 1/5 0]
  Repeating Sequence8 : simulink/Sources/Repeating Sequence  rep_seq_t="[0 (1/fc)/2  (1/fc)]"  rep_seq_y=[1/5 2/5 1/5]
  Repeating Sequence9 : simulink/Sources/Repeating Sequence  rep_seq_t="[0 (1/fc)/2  (1/fc)]"  rep_seq_y=[2/5 3/5 2/5]
  Saturation : Saturate  UpperLimit=1  LowerLimit=0
  Saturation1 : Saturate  UpperLimit=1  LowerLimit=0
  Subsystem : Subsystem
  Sum : Sum  Inputs=-
  Sum1 : Sum  Inputs=-
  Sum2 : Sum
  tag scope: e=global, f=global
  wires:
  Relational Operator10/1 -> [e], [f]
  Sum2/1 -> Relational Operator10/2
  Repeating Sequence10/1 -> Relational Operator10/1
  Saturation/1 -> Sum2/2
  Saturation1/1 -> Sum2/1
  Sum1/1 -> Saturation1/1
  Logical Operator8/1 -> Subsystem/11(In11)
  Relay/1 -> Logical Operator8/1
  Logical Operator5/1 -> Subsystem/7(In7)
  Logical Operator3/1 -> Subsystem/4(In4)
  Logical Operator2/1 -> Subsystem/3(In3)
  Logical Operator1/1 -> Subsystem/2(In2)
  Logical Operator/1 -> Subsystem/1(In1)
  Logical Operator7/1 -> Subsystem/9(In9)
  Logical Operator6/1 -> Subsystem/8(In8)
  Logical Operator4/1 -> Subsystem/6(In6)
  Relational Operator3/1 -> Logical Operator7/2, Subsystem/10(In10)
  Relational Operator2/1 -> Logical Operator6/2, Logical Operator7/1
  Relational Operator9/1 -> Logical Operator5/2, Logical Operator6/1
  Relational Operator8/1 -> Logical Operator4/2, Logical Operator5/1
  Relational Operator7/1 -> Logical Operator4/1, Logical Operator8/2
  Sum/1 -> Relational Operator2/2, Relational Operator3/2, Relational Operator9/2, Relational Operator8/2, Relational Operator7/2, Relay/1
  Repeating Sequence7/1 -> Relational Operator7/1
  Repeating Sequence8/1 -> Relational Operator8/1
  Repeating Sequence9/1 -> Relational Operator9/1
  Repeating Sequence2/1 -> Relational Operator2/1
  Repeating Sequence3/1 -> Relational Operator3/1
  Relational Operator1/1 -> Logical Operator3/2, Subsystem/5(In5)
  Relational Operator/1 -> Logical Operator2/2, Logical Operator3/1
  Relational Operator6/1 -> Logical Operator1/2, Logical Operator2/1
  Relational Operator5/1 -> Logical Operator/2, Logical Operator1/1
  Relational Operator4/1 -> Logical Operator/1
  R1/1(Out1) -> Relational Operator/2, Relational Operator1/2, Relational Operator6/2, Relational Operator5/2, Relational Operator4/2, Sum/1, Saturation/1, Sum1/1
  Repeating Sequence4/1 -> Relational Operator4/1
  Repeating Sequence5/1 -> Relational Operator5/1
  Repeating Sequence6/1 -> Relational Operator6/1
  Repeating Sequence/1 -> Relational Operator/1
  Repeating Sequence1/1 -> Relational Operator1/1

== system latesttopology1/Subsystem4/Subsystem1/PULSE/R1 ==
  Sine Wave : Sin  Amplitude=m  Frequency=2*pi*50  SampleTime=0
  Out1 : Outport
  wires:
  Sine Wave/1 -> Out1/1

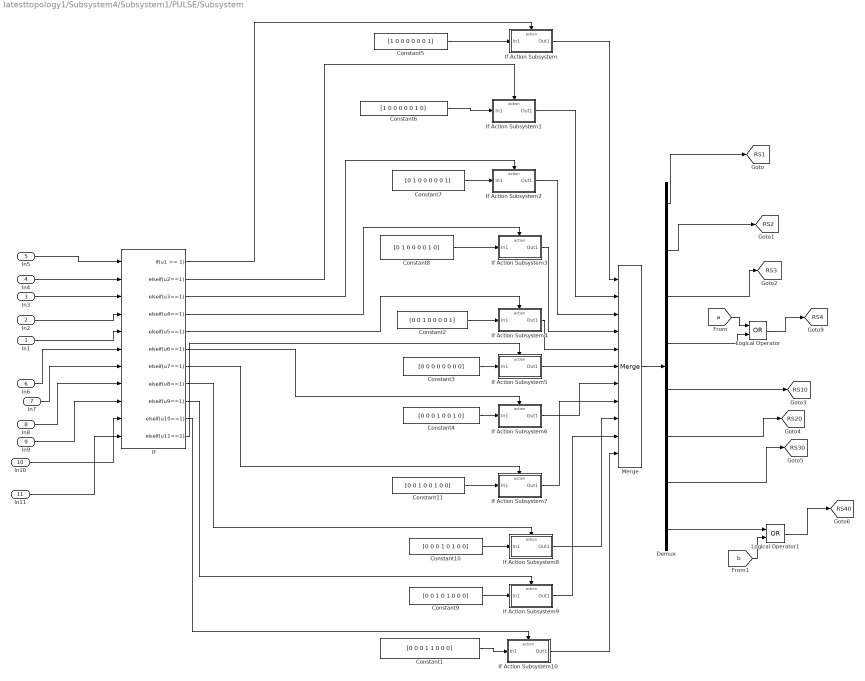
== system latesttopology1/Subsystem4/Subsystem1/PULSE/Subsystem ==
  In1 : Inport
  In2 : Inport  Port=2
  In3 : Inport  Port=3
  In4 : Inport  Port=4
  In5 : Inport  Port=5
  In6 : Inport  Port=6
  In7 : Inport  Port=7
  In8 : Inport  Port=8
  In9 : Inport  Port=9
  In10 : Inport  Port=10
  In11 : Inport  Port=11
  Constant1 : Constant  Value=[0 0 0 1 1 0 0 0]
  Constant10 : Constant  Value=[0 0 0 1 0 1 0 0]
  Constant11 : Constant  Value=[0 0 1 0 0 1 0 0]
  Constant2 : Constant  Value=[0 0 1 0 0 0 0 1]
  Constant3 : Constant  Value=[0 0 0 0 0 0 0 0]
  Constant4 : Constant  Value=[0 0 0 1 0 0 1 0]
  Constant5 : Constant  Value=[1 0 0 0 0 0 0 1]
  Constant6 : Constant  Value=[1 0 0 0 0 0 1 0]
  Constant7 : Constant  Value=[0 1 0 0 0 0 0 1]
  Constant8 : Constant  Value=[0 1 0 0 0 0 1 0]
  Constant9 : Constant  Value=[0 0 1 0 1 0 0 0]
  Demux : Demux  Outputs=8
  If : If  NumInputs=11  IfExpression=u1 == 1  ElseIfExpressions=u2==1, u3==1, u4==1, u5==1, u6==1, u7==1, u8==1, u9==1, u10==1,u11==1  ShowElse=off
  If Action Subsystem : Subsystem  TreatAsAtomicUnit=on
  If Action Subsystem1 : Subsystem  TreatAsAtomicUnit=on
  If Action Subsystem10 : Subsystem  TreatAsAtomicUnit=on
  If Action Subsystem2 : Subsystem  TreatAsAtomicUnit=on
  If Action Subsystem3 : Subsystem  TreatAsAtomicUnit=on
  If Action Subsystem4 : Subsystem  TreatAsAtomicUnit=on
  If Action Subsystem5 : Subsystem  TreatAsAtomicUnit=on
  If Action Subsystem6 : Subsystem  TreatAsAtomicUnit=on
  If Action Subsystem7 : Subsystem  TreatAsAtomicUnit=on
  If Action Subsystem8 : Subsystem  TreatAsAtomicUnit=on
  If Action Subsystem9 : Subsystem  TreatAsAtomicUnit=on
  Logical Operator : Logic  Operator=OR  AllPortsSameDT=off  OutDataTypeStr=boolean
  Logical Operator1 : Logic  Operator=OR  AllPortsSameDT=off  OutDataTypeStr=boolean
  Merge : Merge  Inputs=11
  tag scope: RS10=global, RS1=global, RS20=global, RS2=global, RS30=global, RS3=global, RS40=global, RS4=global
  wires:
  Merge/1 -> Demux/1
  If Action Subsystem/1(Out1) -> Merge/1
  Constant4/1 -> If Action Subsystem6/1(In1)
  Constant3/1 -> If Action Subsystem5/1(In1)
  Constant2/1 -> If Action Subsystem4/1(In1)
  If Action Subsystem1/1(Out1) -> Merge/2
  If Action Subsystem2/1(Out1) -> Merge/3
  If Action Subsystem3/1(Out1) -> Merge/4
  If Action Subsystem4/1(Out1) -> Merge/5
  If Action Subsystem5/1(Out1) -> Merge/6
  If Action Subsystem6/1(Out1) -> Merge/7
  Constant9/1 -> If Action Subsystem9/1(In1)
  Constant10/1 -> If Action Subsystem8/1(In1)
  Constant11/1 -> If Action Subsystem7/1(In1)
  If Action Subsystem10/1(Out1) -> Merge/11
  Constant6/1 -> If Action Subsystem1/1(In1)
  Constant7/1 -> If Action Subsystem2/1(In1)
  Constant8/1 -> If Action Subsystem3/1(In1)
  If Action Subsystem7/1(Out1) -> Merge/8
  If Action Subsystem8/1(Out1) -> Merge/9
  If Action Subsystem9/1(Out1) -> Merge/10
  Demux/3 -> [RS3]
  Demux/2 -> [RS2]
  Demux/1 -> [RS1]
  Constant1/1 -> If Action Subsystem10/1(In1)
  Constant5/1 -> If Action Subsystem/1(In1)
  Demux/5 -> [RS10]
  Demux/6 -> [RS20]
  Demux/7 -> [RS30]
  In5/1 -> If/1
  In4/1 -> If/2
  In3/1 -> If/3
  In2/1 -> If/4
  In1/1 -> If/5
  In10/1 -> If/10
  If/1 -> If Action Subsystem/Action
  If/2 -> If Action Subsystem1/Action
  If/3 -> If Action Subsystem2/Action
  If/4 -> If Action Subsystem3/Action
  If/5 -> If Action Subsystem4/Action
  In9/1 -> If/9
  In8/1 -> If/8
  In7/1 -> If/7
  In6/1 -> If/6
  If/6 -> If Action Subsystem6/Action
  If/7 -> If Action Subsystem7/Action
  If/8 -> If Action Subsystem8/Action
  If/9 -> If Action Subsystem9/Action
  If/10 -> If Action Subsystem10/Action
  If/11 -> If Action Subsystem5/Action
  In11/1 -> If/11
  [a] -> Logical Operator/1
  Demux/4 -> Logical Operator/2
  Logical Operator/1 -> [RS4]
  [b] -> Logical Operator1/2
  Demux/8 -> Logical Operator1/1
  Logical Operator1/1 -> [RS40]

== system latesttopology1/Subsystem4/Subsystem2/PULSE/R1 ==
  Sine Wave : Sin  Amplitude=m  Frequency=2*pi*50  SampleTime=0
  Transport Delay : TransportDelay  DelayTime=(2/3)*0.01
  Out1 : Outport
  wires:
  Sine Wave/1 -> Transport Delay/1
  Transport Delay/1 -> Out1/1

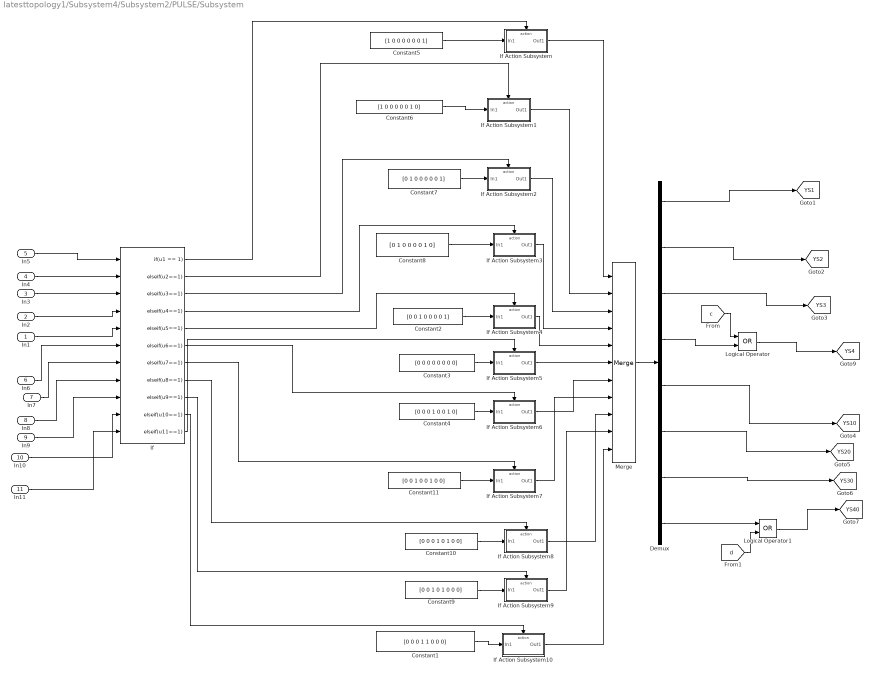
== system latesttopology1/Subsystem4/Subsystem2/PULSE/Subsystem ==
  In1 : Inport
  In2 : Inport  Port=2
  In3 : Inport  Port=3
  In4 : Inport  Port=4
  In5 : Inport  Port=5
  In6 : Inport  Port=6
  In7 : Inport  Port=7
  In8 : Inport  Port=8
  In9 : Inport  Port=9
  In10 : Inport  Port=10
  In11 : Inport  Port=11
  Constant1 : Constant  Value=[0 0 0 1 1 0 0 0]
  Constant10 : Constant  Value=[0 0 0 1 0 1 0 0]
  Constant11 : Constant  Value=[0 0 1 0 0 1 0 0]
  Constant2 : Constant  Value=[0 0 1 0 0 0 0 1]
  Constant3 : Constant  Value=[0 0 0 0 0 0 0 0]
  Constant4 : Constant  Value=[0 0 0 1 0 0 1 0]
  Constant5 : Constant  Value=[1 0 0 0 0 0 0 1]
  Constant6 : Constant  Value=[1 0 0 0 0 0 1 0]
  Constant7 : Constant  Value=[0 1 0 0 0 0 0 1]
  Constant8 : Constant  Value=[0 1 0 0 0 0 1 0]
  Constant9 : Constant  Value=[0 0 1 0 1 0 0 0]
  Demux : Demux  Outputs=8
  If : If  NumInputs=11  IfExpression=u1 == 1  ElseIfExpressions=u2==1, u3==1, u4==1, u5==1, u6==1, u7==1, u8==1, u9==1, u10==1,u11==1  ShowElse=off
  If Action Subsystem : Subsystem  TreatAsAtomicUnit=on
  If Action Subsystem1 : Subsystem  TreatAsAtomicUnit=on
  If Action Subsystem10 : Subsystem  TreatAsAtomicUnit=on
  If Action Subsystem2 : Subsystem  TreatAsAtomicUnit=on
  If Action Subsystem3 : Subsystem  TreatAsAtomicUnit=on
  If Action Subsystem4 : Subsystem  TreatAsAtomicUnit=on
  If Action Subsystem5 : Subsystem  TreatAsAtomicUnit=on
  If Action Subsystem6 : Subsystem  TreatAsAtomicUnit=on
  If Action Subsystem7 : Subsystem  TreatAsAtomicUnit=on
  If Action Subsystem8 : Subsystem  TreatAsAtomicUnit=on
  If Action Subsystem9 : Subsystem  TreatAsAtomicUnit=on
  Logical Operator : Logic  Operator=OR  AllPortsSameDT=off  OutDataTypeStr=boolean
  Logical Operator1 : Logic  Operator=OR  AllPortsSameDT=off  OutDataTypeStr=boolean
  Merge : Merge  Inputs=11
  tag scope: YS10=global, YS1=global, YS20=global, YS2=global, YS30=global, YS3=global, YS40=global, YS4=global
  wires:
  Demux/8 -> Logical Operator1/1
  [d] -> Logical Operator1/2
  Demux/4 -> Logical Operator/2
  [c] -> Logical Operator/1
  In11/1 -> If/11
  If/11 -> If Action Subsystem5/Action
  If/10 -> If Action Subsystem10/Action
  If/9 -> If Action Subsystem9/Action
  If/8 -> If Action Subsystem8/Action
  If/7 -> If Action Subsystem7/Action
  If/6 -> If Action Subsystem6/Action
  In6/1 -> If/6
  In7/1 -> If/7
  In8/1 -> If/8
  In9/1 -> If/9
  If/5 -> If Action Subsystem4/Action
  If/4 -> If Action Subsystem3/Action
  If/3 -> If Action Subsystem2/Action
  If/2 -> If Action Subsystem1/Action
  If/1 -> If Action Subsystem/Action
  In10/1 -> If/10
  In1/1 -> If/5
  In2/1 -> If/4
  In3/1 -> If/3
  In4/1 -> If/2
  In5/1 -> If/1
  Constant5/1 -> If Action Subsystem/1(In1)
  Constant1/1 -> If Action Subsystem10/1(In1)
  If Action Subsystem9/1(Out1) -> Merge/10
  If Action Subsystem8/1(Out1) -> Merge/9
  If Action Subsystem7/1(Out1) -> Merge/8
  Constant8/1 -> If Action Subsystem3/1(In1)
  Constant7/1 -> If Action Subsystem2/1(In1)
  Constant6/1 -> If Action Subsystem1/1(In1)
  If Action Subsystem10/1(Out1) -> Merge/11
  Constant11/1 -> If Action Subsystem7/1(In1)
  Constant10/1 -> If Action Subsystem8/1(In1)
  Constant9/1 -> If Action Subsystem9/1(In1)
  If Action Subsystem6/1(Out1) -> Merge/7
  If Action Subsystem5/1(Out1) -> Merge/6
  If Action Subsystem4/1(Out1) -> Merge/5
  If Action Subsystem3/1(Out1) -> Merge/4
  If Action Subsystem2/1(Out1) -> Merge/3
  If Action Subsystem1/1(Out1) -> Merge/2
  Constant2/1 -> If Action Subsystem4/1(In1)
  Constant3/1 -> If Action Subsystem5/1(In1)
  Constant4/1 -> If Action Subsystem6/1(In1)
  If Action Subsystem/1(Out1) -> Merge/1
  Merge/1 -> Demux/1
  Demux/1 -> [YS1]
  Demux/2 -> [YS2]
  Demux/3 -> [YS3]
  Logical Operator/1 -> [YS4]
  Demux/5 -> [YS10]
  Demux/6 -> [YS20]
  Demux/7 -> [YS30]
  Logical Operator1/1 -> [YS40]

== system latesttopology1/Subsystem4/Subsystem3/PULSE1/R1 ==
  Sine Wave : Sin  Amplitude=m  Frequency=2*pi*50  SampleTime=0
  Transport Delay : TransportDelay  DelayTime=(2/3)*0.01
  Transport Delay1 : TransportDelay  DelayTime=(2/3)*0.01
  Out1 : Outport
  wires:
  Sine Wave/1 -> Transport Delay/1
  Transport Delay/1 -> Transport Delay1/1
  Transport Delay1/1 -> Out1/1

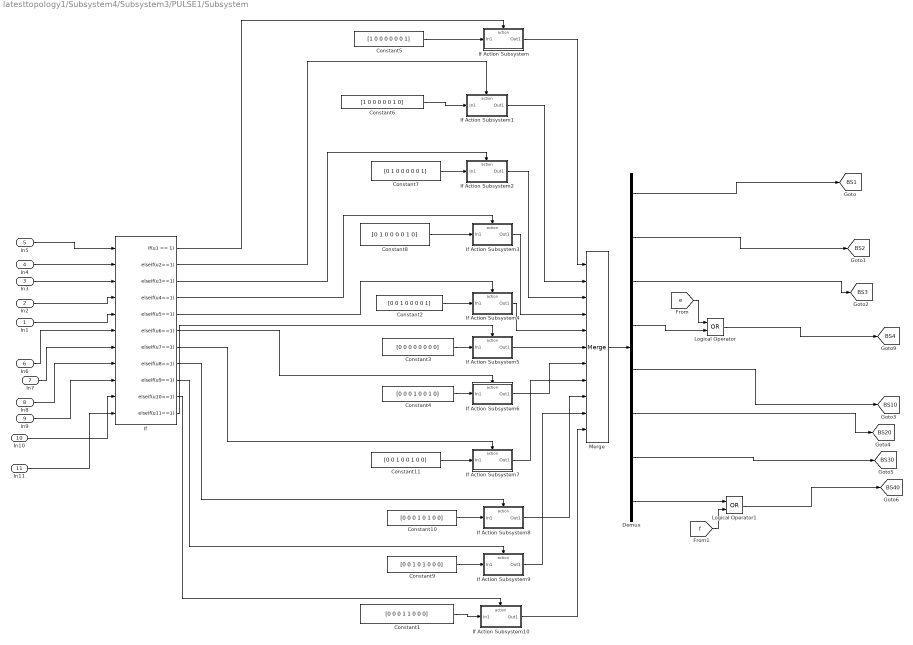
== system latesttopology1/Subsystem4/Subsystem3/PULSE1/Subsystem ==
  In1 : Inport
  In2 : Inport  Port=2
  In3 : Inport  Port=3
  In4 : Inport  Port=4
  In5 : Inport  Port=5
  In6 : Inport  Port=6
  In7 : Inport  Port=7
  In8 : Inport  Port=8
  In9 : Inport  Port=9
  In10 : Inport  Port=10
  In11 : Inport  Port=11
  Constant1 : Constant  Value=[0 0 0 1 1 0 0 0]
  Constant10 : Constant  Value=[0 0 0 1 0 1 0 0]
  Constant11 : Constant  Value=[0 0 1 0 0 1 0 0]
  Constant2 : Constant  Value=[0 0 1 0 0 0 0 1]
  Constant3 : Constant  Value=[0 0 0 0 0 0 0 0]
  Constant4 : Constant  Value=[0 0 0 1 0 0 1 0]
  Constant5 : Constant  Value=[1 0 0 0 0 0 0 1]
  Constant6 : Constant  Value=[1 0 0 0 0 0 1 0]
  Constant7 : Constant  Value=[0 1 0 0 0 0 0 1]
  Constant8 : Constant  Value=[0 1 0 0 0 0 1 0]
  Constant9 : Constant  Value=[0 0 1 0 1 0 0 0]
  Demux : Demux  Outputs=8
  If : If  NumInputs=11  IfExpression=u1 == 1  ElseIfExpressions=u2==1, u3==1, u4==1, u5==1, u6==1, u7==1, u8==1, u9==1, u10==1,u11==1  ShowElse=off
  If Action Subsystem : Subsystem  TreatAsAtomicUnit=on
  If Action Subsystem1 : Subsystem  TreatAsAtomicUnit=on
  If Action Subsystem10 : Subsystem  TreatAsAtomicUnit=on
  If Action Subsystem2 : Subsystem  TreatAsAtomicUnit=on
  If Action Subsystem3 : Subsystem  TreatAsAtomicUnit=on
  If Action Subsystem4 : Subsystem  TreatAsAtomicUnit=on
  If Action Subsystem5 : Subsystem  TreatAsAtomicUnit=on
  If Action Subsystem6 : Subsystem  TreatAsAtomicUnit=on
  If Action Subsystem7 : Subsystem  TreatAsAtomicUnit=on
  If Action Subsystem8 : Subsystem  TreatAsAtomicUnit=on
  If Action Subsystem9 : Subsystem  TreatAsAtomicUnit=on
  Logical Operator : Logic  Operator=OR  AllPortsSameDT=off  OutDataTypeStr=boolean
  Logical Operator1 : Logic  Operator=OR  AllPortsSameDT=off  OutDataTypeStr=boolean
  Merge : Merge  Inputs=11
  tag scope: BS10=global, BS1=global, BS20=global, BS2=global, BS30=global, BS3=global, BS40=global, BS4=global
  wires:
  Demux/8 -> Logical Operator1/1
  [f] -> Logical Operator1/2
  Demux/4 -> Logical Operator/2
  [e] -> Logical Operator/1
  In11/1 -> If/11
  If/11 -> If Action Subsystem5/Action
  If/10 -> If Action Subsystem10/Action
  If/9 -> If Action Subsystem9/Action
  If/8 -> If Action Subsystem8/Action
  If/7 -> If Action Subsystem7/Action
  If/6 -> If Action Subsystem6/Action
  In6/1 -> If/6
  In7/1 -> If/7
  In8/1 -> If/8
  In9/1 -> If/9
  If/5 -> If Action Subsystem4/Action
  If/4 -> If Action Subsystem3/Action
  If/3 -> If Action Subsystem2/Action
  If/2 -> If Action Subsystem1/Action
  If/1 -> If Action Subsystem/Action
  In10/1 -> If/10
  In1/1 -> If/5
  In2/1 -> If/4
  In3/1 -> If/3
  In4/1 -> If/2
  In5/1 -> If/1
  Constant5/1 -> If Action Subsystem/1(In1)
  Constant1/1 -> If Action Subsystem10/1(In1)
  If Action Subsystem9/1(Out1) -> Merge/10
  If Action Subsystem8/1(Out1) -> Merge/9
  If Action Subsystem7/1(Out1) -> Merge/8
  Constant8/1 -> If Action Subsystem3/1(In1)
  Constant7/1 -> If Action Subsystem2/1(In1)
  Constant6/1 -> If Action Subsystem1/1(In1)
  If Action Subsystem10/1(Out1) -> Merge/11
  Constant11/1 -> If Action Subsystem7/1(In1)
  Constant10/1 -> If Action Subsystem8/1(In1)
  Constant9/1 -> If Action Subsystem9/1(In1)
  If Action Subsystem6/1(Out1) -> Merge/7
  If Action Subsystem5/1(Out1) -> Merge/6
  If Action Subsystem4/1(Out1) -> Merge/5
  If Action Subsystem3/1(Out1) -> Merge/4
  If Action Subsystem2/1(Out1) -> Merge/3
  If Action Subsystem1/1(Out1) -> Merge/2
  Constant2/1 -> If Action Subsystem4/1(In1)
  Constant3/1 -> If Action Subsystem5/1(In1)
  Constant4/1 -> If Action Subsystem6/1(In1)
  If Action Subsystem/1(Out1) -> Merge/1
  Merge/1 -> Demux/1
  Demux/3 -> [BS3]
  Demux/2 -> [BS2]
  Demux/1 -> [BS1]
  Logical Operator/1 -> [BS4]
  Demux/5 -> [BS10]
  Demux/6 -> [BS20]
  Demux/7 -> [BS30]
  Logical Operator1/1 -> [BS40]

== system latesttopology1/Subsystem4/Subsystem1/PULSE/Subsystem/If Action Subsystem ==
  In1 : Inport
  Action Port : ActionPort  ActionType=then
  Out1 : Outport
  wires:
  In1/1 -> Out1/1

== system latesttopology1/Subsystem4/Subsystem1/PULSE/Subsystem/If Action Subsystem1 ==
  In1 : Inport
  Action Port : ActionPort  ActionType=elseif
  Out1 : Outport
  wires:
  In1/1 -> Out1/1

== system latesttopology1/Subsystem4/Subsystem1/PULSE/Subsystem/If Action Subsystem10 ==
  In1 : Inport
  Action Port : ActionPort  ActionType=elseif
  Out1 : Outport
  wires:
  In1/1 -> Out1/1

== system latesttopology1/Subsystem4/Subsystem1/PULSE/Subsystem/If Action Subsystem2 ==
  In1 : Inport
  Action Port : ActionPort  ActionType=elseif
  Out1 : Outport
  wires:
  In1/1 -> Out1/1

== system latesttopology1/Subsystem4/Subsystem1/PULSE/Subsystem/If Action Subsystem3 ==
  In1 : Inport
  Action Port : ActionPort  ActionType=elseif
  Out1 : Outport
  wires:
  In1/1 -> Out1/1

== system latesttopology1/Subsystem4/Subsystem1/PULSE/Subsystem/If Action Subsystem4 ==
  In1 : Inport
  Action Port : ActionPort  ActionType=elseif
  Out1 : Outport
  wires:
  In1/1 -> Out1/1

== system latesttopology1/Subsystem4/Subsystem1/PULSE/Subsystem/If Action Subsystem5 ==
  In1 : Inport
  Action Port : ActionPort  ActionType=elseif
  Out1 : Outport
  wires:
  In1/1 -> Out1/1

== system latesttopology1/Subsystem4/Subsystem1/PULSE/Subsystem/If Action Subsystem6 ==
  In1 : Inport
  Action Port : ActionPort  ActionType=elseif
  Out1 : Outport
  wires:
  In1/1 -> Out1/1

== system latesttopology1/Subsystem4/Subsystem1/PULSE/Subsystem/If Action Subsystem7 ==
  In1 : Inport
  Action Port : ActionPort  ActionType=elseif
  Out1 : Outport
  wires:
  In1/1 -> Out1/1

== system latesttopology1/Subsystem4/Subsystem1/PULSE/Subsystem/If Action Subsystem8 ==
  In1 : Inport
  Action Port : ActionPort  ActionType=elseif
  Out1 : Outport
  wires:
  In1/1 -> Out1/1

== system latesttopology1/Subsystem4/Subsystem1/PULSE/Subsystem/If Action Subsystem9 ==
  In1 : Inport
  Action Port : ActionPort  ActionType=elseif
  Out1 : Outport
  wires:
  In1/1 -> Out1/1

== system latesttopology1/Subsystem4/Subsystem2/PULSE/Subsystem/If Action Subsystem ==
  In1 : Inport
  Action Port : ActionPort  ActionType=then
  Out1 : Outport
  wires:
  In1/1 -> Out1/1

== system latesttopology1/Subsystem4/Subsystem2/PULSE/Subsystem/If Action Subsystem1 ==
  In1 : Inport
  Action Port : ActionPort  ActionType=elseif
  Out1 : Outport
  wires:
  In1/1 -> Out1/1

== system latesttopology1/Subsystem4/Subsystem2/PULSE/Subsystem/If Action Subsystem10 ==
  In1 : Inport
  Action Port : ActionPort  ActionType=elseif
  Out1 : Outport
  wires:
  In1/1 -> Out1/1

== system latesttopology1/Subsystem4/Subsystem2/PULSE/Subsystem/If Action Subsystem2 ==
  In1 : Inport
  Action Port : ActionPort  ActionType=elseif
  Out1 : Outport
  wires:
  In1/1 -> Out1/1

== system latesttopology1/Subsystem4/Subsystem2/PULSE/Subsystem/If Action Subsystem3 ==
  In1 : Inport
  Action Port : ActionPort  ActionType=elseif
  Out1 : Outport
  wires:
  In1/1 -> Out1/1

== system latesttopology1/Subsystem4/Subsystem2/PULSE/Subsystem/If Action Subsystem4 ==
  In1 : Inport
  Action Port : ActionPort  ActionType=elseif
  Out1 : Outport
  wires:
  In1/1 -> Out1/1

== system latesttopology1/Subsystem4/Subsystem2/PULSE/Subsystem/If Action Subsystem5 ==
  In1 : Inport
  Action Port : ActionPort  ActionType=elseif
  Out1 : Outport
  wires:
  In1/1 -> Out1/1

== system latesttopology1/Subsystem4/Subsystem2/PULSE/Subsystem/If Action Subsystem6 ==
  In1 : Inport
  Action Port : ActionPort  ActionType=elseif
  Out1 : Outport
  wires:
  In1/1 -> Out1/1

== system latesttopology1/Subsystem4/Subsystem2/PULSE/Subsystem/If Action Subsystem7 ==
  In1 : Inport
  Action Port : ActionPort  ActionType=elseif
  Out1 : Outport
  wires:
  In1/1 -> Out1/1

== system latesttopology1/Subsystem4/Subsystem2/PULSE/Subsystem/If Action Subsystem8 ==
  In1 : Inport
  Action Port : ActionPort  ActionType=elseif
  Out1 : Outport
  wires:
  In1/1 -> Out1/1

== system latesttopology1/Subsystem4/Subsystem2/PULSE/Subsystem/If Action Subsystem9 ==
  In1 : Inport
  Action Port : ActionPort  ActionType=elseif
  Out1 : Outport
  wires:
  In1/1 -> Out1/1

== system latesttopology1/Subsystem4/Subsystem3/PULSE1/Subsystem/If Action Subsystem ==
  In1 : Inport
  Action Port : ActionPort  ActionType=then
  Out1 : Outport
  wires:
  In1/1 -> Out1/1

== system latesttopology1/Subsystem4/Subsystem3/PULSE1/Subsystem/If Action Subsystem1 ==
  In1 : Inport
  Action Port : ActionPort  ActionType=elseif
  Out1 : Outport
  wires:
  In1/1 -> Out1/1

== system latesttopology1/Subsystem4/Subsystem3/PULSE1/Subsystem/If Action Subsystem10 ==
  In1 : Inport
  Action Port : ActionPort  ActionType=elseif
  Out1 : Outport
  wires:
  In1/1 -> Out1/1

== system latesttopology1/Subsystem4/Subsystem3/PULSE1/Subsystem/If Action Subsystem2 ==
  In1 : Inport
  Action Port : ActionPort  ActionType=elseif
  Out1 : Outport
  wires:
  In1/1 -> Out1/1

== system latesttopology1/Subsystem4/Subsystem3/PULSE1/Subsystem/If Action Subsystem3 ==
  In1 : Inport
  Action Port : ActionPort  ActionType=elseif
  Out1 : Outport
  wires:
  In1/1 -> Out1/1

== system latesttopology1/Subsystem4/Subsystem3/PULSE1/Subsystem/If Action Subsystem4 ==
  In1 : Inport
  Action Port : ActionPort  ActionType=elseif
  Out1 : Outport
  wires:
  In1/1 -> Out1/1

== system latesttopology1/Subsystem4/Subsystem3/PULSE1/Subsystem/If Action Subsystem5 ==
  In1 : Inport
  Action Port : ActionPort  ActionType=elseif
  Out1 : Outport
  wires:
  In1/1 -> Out1/1

== system latesttopology1/Subsystem4/Subsystem3/PULSE1/Subsystem/If Action Subsystem6 ==
  In1 : Inport
  Action Port : ActionPort  ActionType=elseif
  Out1 : Outport
  wires:
  In1/1 -> Out1/1

== system latesttopology1/Subsystem4/Subsystem3/PULSE1/Subsystem/If Action Subsystem7 ==
  In1 : Inport
  Action Port : ActionPort  ActionType=elseif
  Out1 : Outport
  wires:
  In1/1 -> Out1/1

== system latesttopology1/Subsystem4/Subsystem3/PULSE1/Subsystem/If Action Subsystem8 ==
  In1 : Inport
  Action Port : ActionPort  ActionType=elseif
  Out1 : Outport
  wires:
  In1/1 -> Out1/1

== system latesttopology1/Subsystem4/Subsystem3/PULSE1/Subsystem/If Action Subsystem9 ==
  In1 : Inport
  Action Port : ActionPort  ActionType=elseif
  Out1 : Outport
  wires:
  In1/1 -> Out1/1
